simulink model "InvertedPendulum"  (R2020a)
settings: Solver=VariableStepAuto  StartTime=0.0  StopTime=50  FixedStep=0.02  RelTol=1e-3
libraries: ctsmodel x1
settings Model: Creator=10564  LastModifiedBy=10564

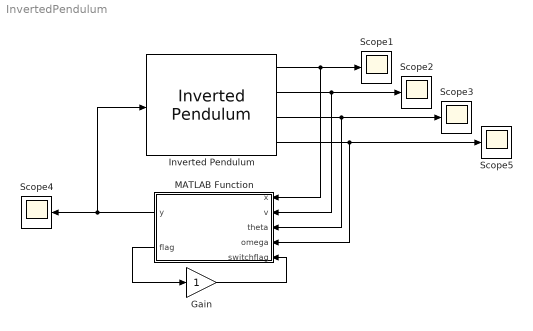
== system InvertedPendulum ==
  Gain : Gain
  Inverted Pendulum : ctsmodel/Inverted Pendulum/Inverted Pendulum  Mc=1  Mp=0.2  L=0.2  Kp=0  Kc=0.1  x=0.1  theta=pi
      settings: SourceProductName=Control System Model Toolbox
  MATLAB Function : MATLAB Function  TreatAsAtomicUnit=on
  Scope{1..5} (5 alike) : Scope
  wires:
  Inverted Pendulum/1 -> MATLAB Function/1(x), Scope1/1
  Inverted Pendulum/2 -> MATLAB Function/2(v), Scope2/1
  Inverted Pendulum/3 -> MATLAB Function/3(theta), Scope3/1
  Inverted Pendulum/4 -> MATLAB Function/4(omega), Scope5/1
  MATLAB Function/1(y) -> Scope4/1, Inverted Pendulum/1
  MATLAB Function/2(flag) -> Gain/1
  Gain/1 -> MATLAB Function/5(switchflag)

== matlab function InvertedPendulum/MATLAB Function ==
  data: x input; y output; v input; theta input; omega input; switchflag input; flag output
function [y,flag] = control(x,v,theta,omega,switchflag)

% model parameters
m = 0.2;
M = 1;
L = 0.2;
g = 9.81;

% Lyapunov control parameters
kv = 1;
kx = 0.01;
kd = 1;
ke = 1;

% LQR K 
K = [-10.0000  -13.9080  -57.6004   -8.0008];

% system energy
E = 0.5*[v,omega]*[m+M m*L*cos(theta);m*L*cos(theta) m*L^2]*[v;omega]+m*g*L*(cos(theta)-1);

% switch to LQR control when approximate to stable point
if (abs(x) < 0.1 && abs(v) < 0.2 && abs(theta) < 0.2 && abs(omega) < 0.1) || (switchflag == 1) 
    y = -K*[x; v; theta; omega]; %LQR
    flag = 1;
else
    flag = 0;
    y = (kv*m*sin(theta)*(g*cos(theta)-L*omega^2)-(M+m*sin(theta)^2)*(kx*x+kd*v))/(kv+(M+m*sin(theta)^2)*ke*E); %Lyapunov
end
